simulink model "DisertatieVanca_Harness1"  (R2022b)
settings: Solver=VariableStepAuto  StartTime=0.0  StopTime=10.0  RelTol=1e-3
settings Model: Creator=uiv66426  LastModifiedBy=uiv66426
settings DebuggingCC: ParameterOverflowMsg=none  ParameterUnderflowMsg=error  ParameterPrecisionLossMsg=none

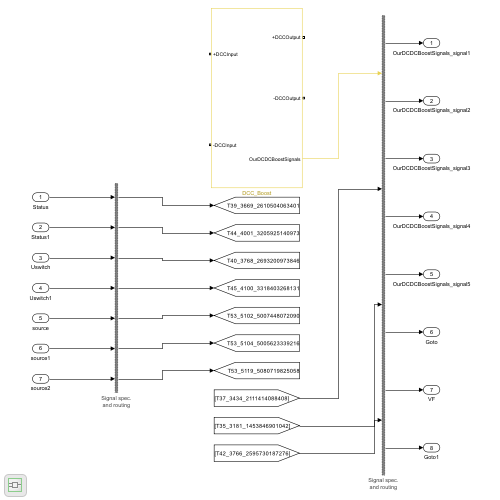
[thumbnail: Simulink's stored preview of the top-level diagram]
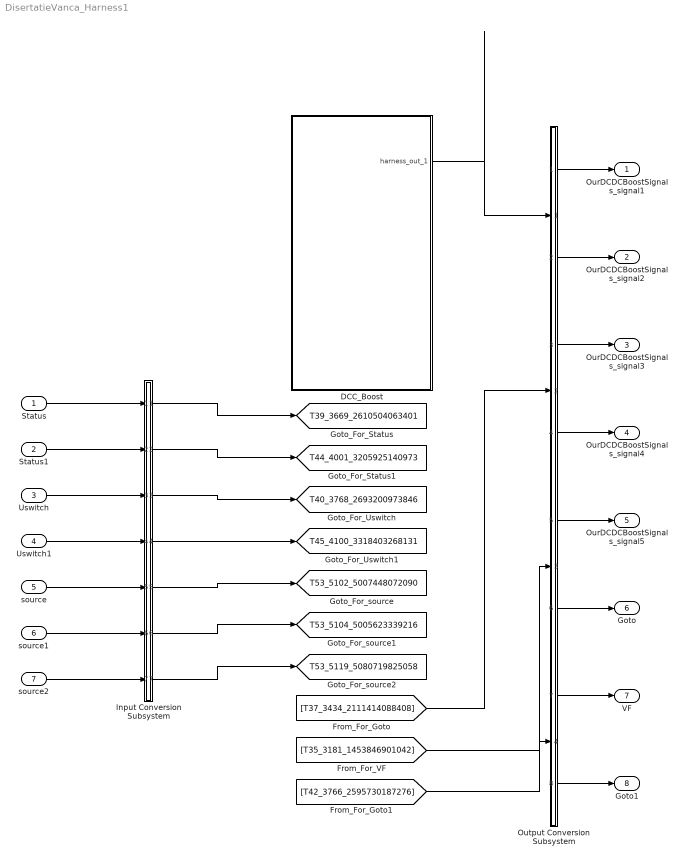
== system DisertatieVanca_Harness1 ==
  Status : Inport  OutDataTypeStr=double  PortDimensions=[1]  SampleTime=5e-05
  Status1 : Inport  Port=2  OutDataTypeStr=double  PortDimensions=[1]  SampleTime=5e-05
  Uswitch : Inport  Port=3  OutDataTypeStr=double  PortDimensions=[1]  SampleTime=5e-05
  Uswitch1 : Inport  Port=4  OutDataTypeStr=double  PortDimensions=[1]  SampleTime=5e-05
  source : Inport  Port=5  OutDataTypeStr=double  PortDimensions=[1]  SampleTime=5e-05
  source1 : Inport  Port=6  OutDataTypeStr=double  PortDimensions=[1]  SampleTime=5e-05
  source2 : Inport  Port=7  OutDataTypeStr=double  PortDimensions=[1]  SampleTime=5e-05
  DCC_Boost : Subsystem  Tag=__SL_testing_harness_stub_
  Input Conversion Subsystem : Subsystem  Tag=__SLT_ICS__  Description=|
      | Signal spec.
      | and routing
      settings: AttributesFormatString=%<Description>
  Output Conversion Subsystem : Subsystem  Tag=__SLT_OCS__  Description=|
      | Signal spec.
      | and routing
      settings: AttributesFormatString=%<Description>
  OurDCDCBoostSignals_signal1 : Outport
  OurDCDCBoostSignals_signal2 : Outport  Port=2
  OurDCDCBoostSignals_signal3 : Outport  Port=3
  OurDCDCBoostSignals_signal4 : Outport  Port=4
  OurDCDCBoostSignals_signal5 : Outport  Port=5
  Goto : Outport  Port=6
  VF : Outport  Port=7
  Goto1 : Outport  Port=8
  tag scope: T39_3669_2610504063401=global, T40_3768_2693200973846=global, T44_4001_3205925140973=global, T45_4100_3318403268131=global, T53_5102_5007448072090=global, T53_5104_5005623339216=global, T53_5119_5080719825058=global
  wires:
  Status/1 -> Input Conversion Subsystem/1(Inport_1)
  Status1/1 -> Input Conversion Subsystem/2(Inport_2)
  Uswitch/1 -> Input Conversion Subsystem/3(Inport_3)
  Uswitch1/1 -> Input Conversion Subsystem/4(Inport_4)
  source/1 -> Input Conversion Subsystem/5(Inport_5)
  source1/1 -> Input Conversion Subsystem/6(Inport_6)
  source2/1 -> Input Conversion Subsystem/7(Inport_7)
  Output Conversion Subsystem/1(Outport_1) -> OurDCDCBoostSignals_signal1/1
  Output Conversion Subsystem/2(Outport_2) -> OurDCDCBoostSignals_signal2/1
  Output Conversion Subsystem/3(Outport_3) -> OurDCDCBoostSignals_signal3/1
  Output Conversion Subsystem/4(Outport_4) -> OurDCDCBoostSignals_signal4/1
  Output Conversion Subsystem/5(Outport_5) -> OurDCDCBoostSignals_signal5/1
  Output Conversion Subsystem/6(Outport_6) -> Goto/1
  Output Conversion Subsystem/7(Outport_7) -> VF/1
  Output Conversion Subsystem/8(Outport_8) -> Goto1/1
  Input Conversion Subsystem/1(Outport_1) -> [T39_3669_2610504063401]
  Input Conversion Subsystem/2(Outport_2) -> [T44_4001_3205925140973]
  Input Conversion Subsystem/3(Outport_3) -> [T40_3768_2693200973846]
  Input Conversion Subsystem/4(Outport_4) -> [T45_4100_3318403268131]
  Input Conversion Subsystem/5(Outport_5) -> [T53_5102_5007448072090]
  Input Conversion Subsystem/6(Outport_6) -> [T53_5104_5005623339216]
  Input Conversion Subsystem/7(Outport_7) -> [T53_5119_5080719825058]
  DCC_Boost/1(harness_out_1) -> Output Conversion Subsystem/1(Inport_1)
  [T37_3434_2111414088408] -> Output Conversion Subsystem/2(Inport_2)
  [T35_3181_1453846901042] -> Output Conversion Subsystem/3(Inport_3)
  [T42_3766_2595730187276] -> Output Conversion Subsystem/4(Inport_4)

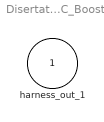
== system DisertatieVanca_Harness1/DCC_Boost ==
  harness_out_1 : Outport

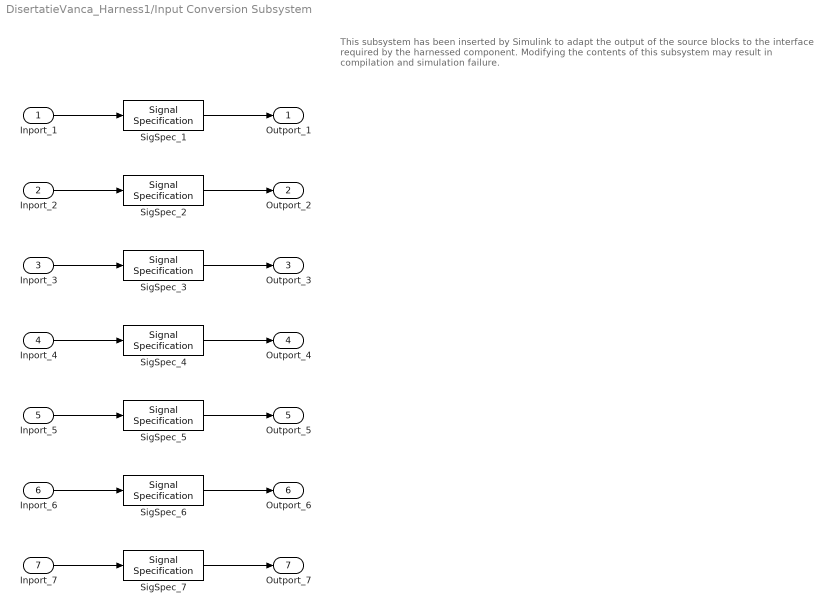
== system DisertatieVanca_Harness1/Input Conversion Subsystem ==
  note: This subsystem has been inserted by Simulink to adapt the output of the source blocks to the interface required by the harnessed component.
      |  Modifying the contents of this subsystem may result in compilation and simulation failure.
  Inport_1 : Inport
  Inport_2 : Inport  Port=2
  Inport_3 : Inport  Port=3
  Inport_4 : Inport  Port=4
  Inport_5 : Inport  Port=5
  Inport_6 : Inport  Port=6
  Inport_7 : Inport  Port=7
  SigSpec_{1..7} (7 alike) : SignalSpecification  OutDataTypeStr=double  Dimensions=[1]  SampleTime=5e-05
  Outport_1 : Outport
  Outport_2 : Outport  Port=2
  Outport_3 : Outport  Port=3
  Outport_4 : Outport  Port=4
  Outport_5 : Outport  Port=5
  Outport_6 : Outport  Port=6
  Outport_7 : Outport  Port=7
  wires:
  SigSpec_1/1 -> Outport_1/1
  Inport_1/1 -> SigSpec_1/1
  SigSpec_2/1 -> Outport_2/1
  Inport_2/1 -> SigSpec_2/1
  SigSpec_3/1 -> Outport_3/1
  Inport_3/1 -> SigSpec_3/1
  SigSpec_4/1 -> Outport_4/1
  Inport_4/1 -> SigSpec_4/1
  SigSpec_5/1 -> Outport_5/1
  Inport_5/1 -> SigSpec_5/1
  SigSpec_6/1 -> Outport_6/1
  Inport_6/1 -> SigSpec_6/1
  SigSpec_7/1 -> Outport_7/1
  Inport_7/1 -> SigSpec_7/1

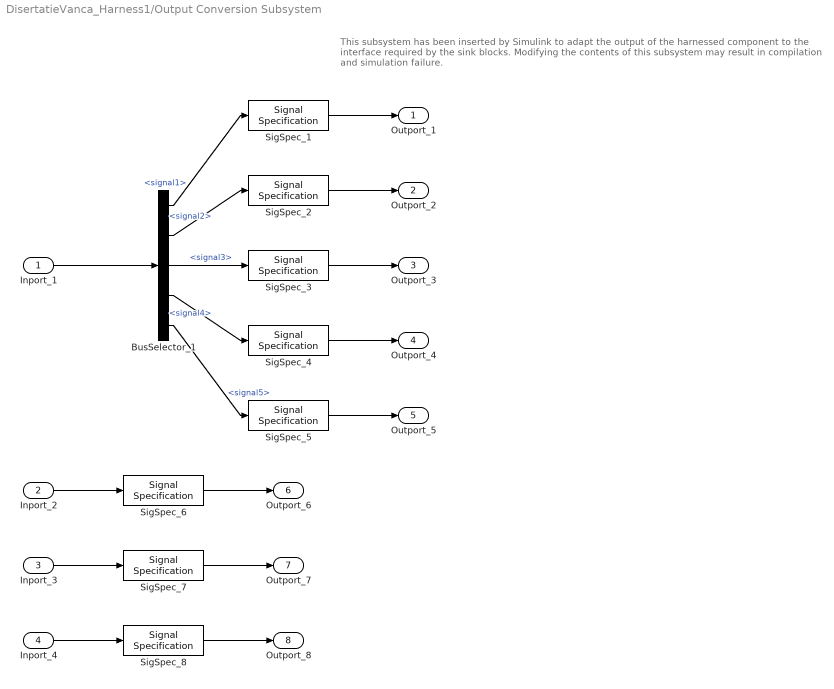
== system DisertatieVanca_Harness1/Output Conversion Subsystem ==
  note: This subsystem has been inserted by Simulink to adapt the output of the harnessed component to the interface required by the sink blocks.
      |  Modifying the contents of this subsystem may result in compilation and simulation failure.
  Inport_1 : Inport
  Inport_2 : Inport  Port=2
  Inport_3 : Inport  Port=3
  Inport_4 : Inport  Port=4
  BusSelector_1 : BusSelector  OutputSignals=signal1,signal2,signal3,signal4,signal5
  SigSpec_1 : SignalSpecification  OutDataTypeStr=double  Dimensions=[1]  SampleTime=5e-05
  SigSpec_2 : SignalSpecification  OutDataTypeStr=double  Dimensions=[1]  SampleTime=5e-05
  SigSpec_{3..4,6..7} (4 alike) : SignalSpecification  OutDataTypeStr=double  Dimensions=[1]
  SigSpec_5 : SignalSpecification  OutDataTypeStr=boolean  Dimensions=[1]  SampleTime=5e-05
  SigSpec_8 : SignalSpecification  OutDataTypeStr=double  Dimensions=[1]  SampleTime=5e-05
  Outport_1 : Outport
  Outport_2 : Outport  Port=2
  Outport_3 : Outport  Port=3
  Outport_4 : Outport  Port=4
  Outport_5 : Outport  Port=5
  Outport_6 : Outport  Port=6
  Outport_7 : Outport  Port=7
  Outport_8 : Outport  Port=8
  wires:
  Inport_1/1 -> BusSelector_1/1
  BusSelector_1/1 -> SigSpec_1/1  "<signal1>"
  SigSpec_1/1 -> Outport_1/1
  BusSelector_1/2 -> SigSpec_2/1  "<signal2>"
  SigSpec_2/1 -> Outport_2/1
  BusSelector_1/3 -> SigSpec_3/1  "<signal3>"
  SigSpec_3/1 -> Outport_3/1
  BusSelector_1/4 -> SigSpec_4/1  "<signal4>"
  SigSpec_4/1 -> Outport_4/1
  BusSelector_1/5 -> SigSpec_5/1  "<signal5>"
  SigSpec_5/1 -> Outport_5/1
  Inport_2/1 -> SigSpec_6/1
  SigSpec_6/1 -> Outport_6/1
  Inport_3/1 -> SigSpec_7/1
  SigSpec_7/1 -> Outport_7/1
  Inport_4/1 -> SigSpec_8/1
  SigSpec_8/1 -> Outport_8/1
